simulink model "satellite3"  (R2025b)
settings: Solver=FixedStepAuto  StartTime=0.0  StopTime=100  FixedStep=dt  MinStep=0.0001  RelTol=1e-3
values from neighbouring files (symbols this model uses):
  A_mw = [ ... (first row only)    [init_params.m]
  A_w = [ ... (first row only)    [init_params.m]
  alpha1 = 0.1    [init_params.m]
  alpha2 = 0.1    [init_params.m]
  angle0 = eAR'    [init_params.m]
  area_d = 4    [init_params.m]
  area_m2 = 0.0127    [init_params.m]
  area_s = 2    [init_params.m]
  ARW_deg_per_sqrt_h = 0.01    [init_params.m]
  B_mw = [ ... (first row only)    [init_params.m]
  bat_bias_on = 0    [init_params.m]
  bat_bias_time = 0    [init_params.m]
  bat_bias_value = 0    [init_params.m]
  bat_cap_on = 0    [init_params.m]
  bat_cap_time = 0    [init_params.m]
  bat_cap_value = 1    [init_params.m]
  beta = 0.3    [init_params.m]
  beta1 = 0.01    [init_params.m]
  beta2 = 0.01    [init_params.m]
  bias0_deg_h = 0.01    [init_params.m]
  C_mw = [ ... (first row only)    [init_params.m]
  Cd = 2.2    [init_params.m]
  Cm = 0.01    [init_params.m]
  cmd_comm = 1    [init_params.m]
  comm_allow = 1    [init_params.m]
  cos_g_max = cos(gamma_max)    [init_params.m]
  Cr = 1.2    [init_params.m]
  cT_deg_on = 0    [init_params.m]
  cT_deg_time = 0    [init_params.m]
  cT_deg_value = 1    [init_params.m]
  cT_delay_on = 0    [init_params.m]
  cT_delay_time = 0    [init_params.m]
  cT_delay_value = 0    [init_params.m]
  cT_drop_on = 0    [init_params.m]
  cT_drop_time = 0    [init_params.m]
  cT_drop_value = 0    [init_params.m]
  cT_lock_on = 0    [init_params.m]
  cT_lock_time = 0    [init_params.m]
  d_c = 2e-5    (= 2e-05)    [init_params.m]
  d_f = 2e-5    (= 2e-05)    [init_params.m]
  D_max = 1    [init_params.m]
  D_thr = 0.4    [init_params.m]
  Delta_D = 0.001    [init_params.m]
  dP_th = 0.05    [init_params.m]
  dss_bias_on = 0    [init_params.m]
  dss_bias_time = 0    [init_params.m]
  dss_bias_value = [0;0;0]    [init_params.m]
  dss_delay_on = 0    [init_params.m]
  dss_delay_time = 0    [init_params.m]
  dss_delay_value = 0    [init_params.m]
  dss_drift_max = 0.1    [init_params.m]
  dss_drift_value = [0;0;0]    [init_params.m]
  dss_drop_on = 0    [init_params.m]
  dss_drop_time = 0    [init_params.m]
  dss_drop_value = [1;0;0]    [init_params.m]
  dss_lock_on = 0    [init_params.m]
  dss_lock_time = 0    [init_params.m]
  dt = 0.1    [init_params.m]
  earth_theta0 = 0    [init_params.m]
  epsilon = 0.01    [init_params.m]
  eT_deg_on = 0    [init_params.m]
  eT_deg_time = 0    [init_params.m]
  eT_deg_value = 1    [init_params.m]
  eT_delay_on = 0    [init_params.m]
  eT_delay_time = 0    [init_params.m]
  eT_delay_value = 0    [init_params.m]
  eT_drop_on = 0    [init_params.m]
  eT_drop_time = 0    [init_params.m]
  eT_drop_value = [0;0;0]    [init_params.m]
  eT_lock_on = 0    [init_params.m]
  eT_lock_time = 0    [init_params.m]
  eta = 0.7    [init_params.m]
  eta_buck = 0.9    [init_params.m]
  eta_et = 0.9    [init_params.m]
  eta_sspa = 0.35    [init_params.m]
  eta_twta = 0.35    [init_params.m]
  f = 2.2e9    (= 2200000000)    [init_params.m]
  f_n_hz = 400    [init_params.m]
  fov = 60*pi/180    (= 1.0471975512)    [init_params.m]
  g0 = 9.80665    [init_params.m]
  G0 = 1366.1    [init_params.m]
  G_sspa_dB = 20    [init_params.m]
  G_twta_dB = 20    [init_params.m]
  Gr_dB = 20    [init_params.m]
  Gt_dB = 3    [init_params.m]
  gyro_bias_on = 0    [init_params.m]
  gyro_bias_time = 0    [init_params.m]
  gyro_bias_value = [0;0;0]    [init_params.m]
  gyro_delay_on = 0    [init_params.m]
  gyro_delay_time = 0    [init_params.m]
  gyro_delay_value = 0    [init_params.m]
  gyro_drift_max = 0.1    [init_params.m]
  gyro_drift_value = [0;0;0]    [init_params.m]
  gyro_drop_on = 0    [init_params.m]
  gyro_drop_time = 0    [init_params.m]
  gyro_drop_value = [0;0;0]    [init_params.m]
  gyro_lock_on = 0    [init_params.m]
  gyro_lock_time = 0    [init_params.m]
  H = 50e3    (= 50000)    [init_params.m]
  h_max = Iw * rpm_max * sqrt(6)    [init_params.m]
  h_ref = 400e3    (= 400000)    [init_params.m]
  I_e = 11    [init_params.m]
  I_gate = 0.5    [init_params.m]
  I_triggle = 8    [init_params.m]
  i_w_max = 2    [init_params.m]
  i_w_min = -2    [init_params.m]
  initial_phase = 0    [init_params.m]
  Isp = 220    [init_params.m]
  Isp_et = 1500    [init_params.m]
  Iw = 0.02    [init_params.m]
  J2 = 1.08262668e-3    (= 0.00108262668)    [init_params.m]
  Jx = 10    [init_params.m]
  Jy = 12    [init_params.m]
  Jz = 8    [init_params.m]
  k_a = 4e-4    (= 0.0004)    [init_params.m]
  k_bias1_deg_h_per_C = 1    [init_params.m]
  k_bias2_deg_h_per_C = 0.0    (= 0)    [init_params.m]
  k_h = -0.05    [init_params.m]
  k_sf1_ppm = 1.0    (= 1)    [init_params.m]
  k_sf2_ppm = 0.0    (= 0)    [init_params.m]
  ... (+207 more)
libraries: matrix_library x25, simulink x14, nesl_utility x4, simulink_extras x3, fl_lib x3, ee_lib x1
(part 4 of 5)

== system satellite3/姿态确定与控制系统/三轴姿态动力学子系统/姿态解算/简化互补滤波器/四元数乘法 ==
  Q1 : Inport
  Q2 : Inport  Port=2
  Add : Sum  Inputs=3
  Cross Product : matrix_library/Cross Product
  Demux : Demux
  Demux1 : Demux
  Dot Product : DotProduct  OutDataTypeStr=Inherit: Inherit via internal rule
  Mux : Mux  Inputs=2
  Mux1 : Mux  Inputs=3
  Mux2 : Mux  Inputs=3
  Product : Product
  Product1 : Product
  Product2 : Product
  Sum : Sum  Inputs=|+-
  Q : Outport
  wires:
  Q1/1 -> Demux/1
  Q2/1 -> Demux1/1
  Mux/1 -> Q/1
  Product/1 -> Sum/1
  Demux/1 -> Product1/1, Product/1
  Mux1/1 -> Dot Product/1, Cross Product/1, Product2/2
  Demux1/1 -> Product2/1, Product/2
  Mux2/1 -> Cross Product/2, Dot Product/2, Product1/2
  Sum/1 -> Mux/1
  Dot Product/1 -> Sum/2
  Product2/1 -> Add/2
  Product1/1 -> Add/1
  Cross Product/1 -> Add/3
  Add/1 -> Mux/2
  Demux/2 -> Mux1/1
  Demux/3 -> Mux1/2
  Demux/4 -> Mux1/3
  Demux1/2 -> Mux2/1
  Demux1/3 -> Mux2/2
  Demux1/4 -> Mux2/3

== system satellite3/姿态确定与控制系统/三轴姿态动力学子系统/姿态解算/简化互补滤波器/四元数传播-欧拉法 ==
  note: $\dot{q}=\frac{1}{2} \left[\begin{array}{ccc} -q_1&-q_2&-q_3 \\ q_0&-q_3&q_2\\ q_3&q_0&-q_1\\ -q_2&q_1&q_0 \end{array}\right]\omega$
  机体系角速度分量 : Inport
  Demux : Demux
  Int_q0 : Integrator  InitialCondition=Q0(1)
  Int_q1 : Integrator  InitialCondition=Q0(2)
  Int_q2 : Integrator  InitialCondition=Q0(3)
  Int_q3 : Integrator  InitialCondition=Q0(4)
  Mux : Mux
  Product : Product  Multiplication=Matrix(*)
  Product{1..4} (4 alike) : Product  Inputs=*/
  Transpose : Math  Operator=transpose
  Vector Concatenate : Concatenate  NumInputs=4  Mode=Multidimensional array  ConcatenateDimension=2
  neg1 : Gain  Gain=-1
  neg2 : Gain  Gain=-1
  neg3 : Gain  Gain=-1
  q0_dot : Mux  Inputs=3
  q1_dot : Mux  Inputs=3
  q1_dot1 : Mux  Inputs=3
  q1_dot2 : Mux  Inputs=3
  向量模长-q : Subsystem
  四元数 : Outport
  wires:
  Product/1 -> Demux/1
  neg1/1 -> q0_dot/1, q1_dot1/3
  q1_dot/1 -> Vector Concatenate/2
  neg3/1 -> q1_dot/2, q0_dot/3
  Product4/1 -> neg3/1, Mux/4, q1_dot1/1  "q3"
  Product1/1 -> q1_dot/1, q1_dot1/2, Mux/1, q1_dot2/3  "q0"
  q1_dot1/1 -> Vector Concatenate/3
  Demux/2 -> Int_q1/1
  Product2/1 -> neg1/1, Mux/2, q1_dot2/2  "q1"
  Demux/3 -> Int_q2/1
  neg2/1 -> q1_dot2/1, q0_dot/2
  q1_dot2/1 -> Vector Concatenate/4
  Product3/1 -> neg2/1, Mux/3, q1_dot/3  "q2"
  q0_dot/1 -> Vector Concatenate/1
  Vector Concatenate/1 -> Transpose/1
  Demux/1 -> Int_q0/1
  Demux/4 -> Int_q3/1
  机体系角速度分量/1 -> Product/2
  Transpose/1 -> Product/1
  Int_q0/1 -> Product1/1, 向量模长-q/1(u0)
  Int_q1/1 -> Product2/1, 向量模长-q/2(u1)
  Int_q2/1 -> Product3/1, 向量模长-q/3(u2)
  Int_q3/1 -> Product4/1, 向量模长-q/4(u3)
  向量模长-q/1(|u|) -> Product2/2, Product3/2, Product4/2, Product1/2
  Mux/1 -> 四元数/1

== system satellite3/姿态确定与控制系统/三轴姿态动力学子系统/姿态解算/简化互补滤波器/太敏&地敏 ==
  note: 可见性：一般只要不被遮挡都能工作；
      | 当高度太高（或地球在传感器背面）判 invalid
  太阳矢量 : Inport
  hat_r_o : Inport  Port=2
  q_hat : Inport  Port=3
  q_true : Inport  Port=4
  Add : Sum
  Cross Product : matrix_library/Cross Product
  Cross Product1 : matrix_library/Cross Product
  Gain : Gain  Gain=0.6
  Gain1 : Gain  Gain=0.4
  地敏测量 : Subsystem
  地敏预测 : Subsystem
  太敏测量 : Subsystem
  太敏预测 : Subsystem
  e_c : Outport
  wires:
  太阳矢量/1 -> 太敏测量/2(太阳矢量), 太敏预测/2(太阳矢量)
  hat_r_o/1 -> 地敏预测/1(hat_r_o), 地敏测量/1(hat_r_o)
  太敏预测/1(s_b_meas) -> Cross Product/1
  太敏测量/1(s_b_meas) -> Cross Product/2
  q_true/1 -> 地敏测量/2(q_true), 太敏测量/1(q_true)
  q_hat/1 -> 太敏预测/1(q_hat), 地敏预测/3(q_hat)
  地敏预测/1(nadir_b_meas) -> Cross Product1/1
  地敏测量/1(nadir_b_meas) -> Cross Product1/2
  Cross Product/1 -> Gain/1
  Cross Product1/1 -> Gain1/1
  Gain/1 -> Add/1
  Gain1/1 -> Add/2
  Add/1 -> e_c/1

== system satellite3/姿态确定与控制系统/三轴姿态动力学子系统/姿态解算/简化互补滤波器/星敏故障 ==
  原值 : Inport
  Add : Sum  Inputs=+++++
  Sum : Sum  Inputs=|++
  偏差故障 : Subsystem
  延迟故障 : Subsystem
  掉线故障 : Subsystem
  漂移故障 : Subsystem
  锁死故障 : Subsystem
  故障值 : Outport
  wires:
  延迟故障/1(故障值注入) -> Add/5
  掉线故障/1(故障值注入) -> Add/4
  锁死故障/1(故障值注入) -> Add/3
  漂移故障/1(故障值注入) -> Add/2
  偏差故障/1(故障值注入) -> Add/1
  Add/1 -> Sum/2
  Sum/1 -> 故障值/1
  原值/1 -> Sum/1, 锁死故障/1(原值), 掉线故障/1(原值), 延迟故障/1(原值)

== system satellite3/姿态确定与控制系统/金字塔反作用轮组件/反作用轮组件/反作用轮1/摩擦模型 ==
  note: Stribeck/死区/轴承复杂摩擦:是真实工程里会做的，但不建议上。因为：
      | 参数难找
      | 容易导致数值振荡
      | 对系统级闭环验证意义不如前两层大
  转速 : Inport
  Add : Sum
  Sign : Signum
  库仑摩擦系数 : Gain  Gain=d_c
  粘性摩擦系数 : Gain  Gain=d_f
  摩擦力矩 : Outport
  wires:
  转速/1 -> 粘性摩擦系数/1, Sign/1
  Sign/1 -> 库仑摩擦系数/1
  库仑摩擦系数/1 -> Add/2
  粘性摩擦系数/1 -> Add/1
  Add/1 -> 摩擦力矩/1

== system satellite3/姿态确定与控制系统/金字塔反作用轮组件/反作用轮组件/反作用轮1/轮力矩故障 ==
  原值 : Inport
  Add : Sum  Inputs=++++++
  Sum : Sum  Inputs=|++
  延迟故障 : Subsystem
  掉线故障 : Subsystem
  迟缓故障 : Subsystem
  退化故障 : Subsystem
  锁死故障 : Subsystem
  饱和故障 : Subsystem
  故障值 : Outport
  wires:
  延迟故障/1(故障值注入) -> Add/3
  饱和故障/1(故障值注入) -> Add/2
  退化故障/1(故障值注入) -> Add/1
  Add/1 -> Sum/2
  Sum/1 -> 故障值/1
  原值/1 -> Sum/1, 锁死故障/1(原值), 迟缓故障/1(原值), 掉线故障/1(原值), 延迟故障/1(原值), 饱和故障/1(原值), 退化故障/1(原值)
  掉线故障/1(故障值注入) -> Add/4
  迟缓故障/1(故障值注入) -> Add/5
  锁死故障/1(故障值注入) -> Add/6

== system satellite3/姿态确定与控制系统/金字塔反作用轮组件/反作用轮组件/反作用轮1/轮摩擦故障 ==
  原值 : Inport
  Add : Sum
  Sum : Sum  Inputs=|++
  乘性故障 : Subsystem
  偏差故障 : Subsystem
  故障值 : Outport
  wires:
  乘性故障/1(故障值注入) -> Add/2
  Sum/1 -> 故障值/1
  原值/1 -> Sum/1, 乘性故障/1(原值)
  偏差故障/1(故障值注入) -> Add/1
  Add/1 -> Sum/2

== system satellite3/姿态确定与控制系统/金字塔反作用轮组件/反作用轮组件/反作用轮1/轮状态解算 ==
  作用力矩 : Inport
  积分得到转速 : Integrator
  转动惯量 : Gain  Gain=Iw
  除以转动惯量 : Gain  Gain=1/Iw
  转速 : Outport
  角动量 : Outport  Port=2
  wires:
  积分得到转速/1 -> 转动惯量/1, 转速/1
  除以转动惯量/1 -> 积分得到转速/1
  作用力矩/1 -> 除以转动惯量/1
  转动惯量/1 -> 角动量/1

== system satellite3/姿态确定与控制系统/金字塔反作用轮组件/反作用轮组件/反作用轮2/摩擦模型 ==
  note: Stribeck/死区/轴承复杂摩擦:是真实工程里会做的，但不建议上。因为：
      | 参数难找
      | 容易导致数值振荡
      | 对系统级闭环验证意义不如前两层大
  转速 : Inport
  Add : Sum
  Sign : Signum
  库仑摩擦系数 : Gain  Gain=d_c
  粘性摩擦系数 : Gain  Gain=d_f
  摩擦力矩 : Outport
  wires:
  Add/1 -> 摩擦力矩/1
  粘性摩擦系数/1 -> Add/1
  库仑摩擦系数/1 -> Add/2
  Sign/1 -> 库仑摩擦系数/1
  转速/1 -> Sign/1, 粘性摩擦系数/1

== system satellite3/姿态确定与控制系统/金字塔反作用轮组件/反作用轮组件/反作用轮2/轮力矩故障 ==
  原值 : Inport
  Add : Sum  Inputs=++++++
  Sum : Sum  Inputs=|++
  延迟故障 : Subsystem
  掉线故障 : Subsystem
  迟缓故障 : Subsystem
  退化故障 : Subsystem
  锁死故障 : Subsystem
  饱和故障 : Subsystem
  故障值 : Outport
  wires:
  锁死故障/1(故障值注入) -> Add/6
  迟缓故障/1(故障值注入) -> Add/5
  掉线故障/1(故障值注入) -> Add/4
  原值/1 -> 退化故障/1(原值), 饱和故障/1(原值), 延迟故障/1(原值), 掉线故障/1(原值), 迟缓故障/1(原值), 锁死故障/1(原值), Sum/1
  Sum/1 -> 故障值/1
  Add/1 -> Sum/2
  退化故障/1(故障值注入) -> Add/1
  饱和故障/1(故障值注入) -> Add/2
  延迟故障/1(故障值注入) -> Add/3

== system satellite3/姿态确定与控制系统/金字塔反作用轮组件/反作用轮组件/反作用轮2/轮摩擦故障 ==
  原值 : Inport
  Add : Sum
  Sum : Sum  Inputs=|++
  乘性故障 : Subsystem
  偏差故障 : Subsystem
  故障值 : Outport
  wires:
  乘性故障/1(故障值注入) -> Add/2
  Sum/1 -> 故障值/1
  原值/1 -> Sum/1, 乘性故障/1(原值)
  偏差故障/1(故障值注入) -> Add/1
  Add/1 -> Sum/2

== system satellite3/姿态确定与控制系统/金字塔反作用轮组件/反作用轮组件/反作用轮2/轮状态解算 ==
  作用力矩 : Inport
  积分得到转速 : Integrator
  转动惯量 : Gain  Gain=Iw
  除以转动惯量 : Gain  Gain=1/Iw
  转速 : Outport
  角动量 : Outport  Port=2
  wires:
  转动惯量/1 -> 角动量/1
  作用力矩/1 -> 除以转动惯量/1
  除以转动惯量/1 -> 积分得到转速/1
  积分得到转速/1 -> 转速/1, 转动惯量/1

== system satellite3/姿态确定与控制系统/金字塔反作用轮组件/反作用轮组件/反作用轮3/摩擦模型 ==
  note: Stribeck/死区/轴承复杂摩擦:是真实工程里会做的，但不建议上。因为：
      | 参数难找
      | 容易导致数值振荡
      | 对系统级闭环验证意义不如前两层大
  转速 : Inport
  Add : Sum
  Sign : Signum
  库仑摩擦系数 : Gain  Gain=d_c
  粘性摩擦系数 : Gain  Gain=d_f
  摩擦力矩 : Outport
  wires:
  转速/1 -> 粘性摩擦系数/1, Sign/1
  Sign/1 -> 库仑摩擦系数/1
  库仑摩擦系数/1 -> Add/2
  粘性摩擦系数/1 -> Add/1
  Add/1 -> 摩擦力矩/1

== system satellite3/姿态确定与控制系统/金字塔反作用轮组件/反作用轮组件/反作用轮3/轮力矩故障 ==
  原值 : Inport
  Add : Sum  Inputs=++++++
  Sum : Sum  Inputs=|++
  延迟故障 : Subsystem
  掉线故障 : Subsystem
  迟缓故障 : Subsystem
  退化故障 : Subsystem
  锁死故障 : Subsystem
  饱和故障 : Subsystem
  故障值 : Outport
  wires:
  延迟故障/1(故障值注入) -> Add/3
  饱和故障/1(故障值注入) -> Add/2
  退化故障/1(故障值注入) -> Add/1
  Add/1 -> Sum/2
  Sum/1 -> 故障值/1
  原值/1 -> Sum/1, 锁死故障/1(原值), 迟缓故障/1(原值), 掉线故障/1(原值), 延迟故障/1(原值), 饱和故障/1(原值), 退化故障/1(原值)
  掉线故障/1(故障值注入) -> Add/4
  迟缓故障/1(故障值注入) -> Add/5
  锁死故障/1(故障值注入) -> Add/6

== system satellite3/姿态确定与控制系统/金字塔反作用轮组件/反作用轮组件/反作用轮3/轮摩擦故障 ==
  原值 : Inport
  Add : Sum
  Sum : Sum  Inputs=|++
  乘性故障 : Subsystem
  偏差故障 : Subsystem
  故障值 : Outport
  wires:
  乘性故障/1(故障值注入) -> Add/2
  Sum/1 -> 故障值/1
  原值/1 -> Sum/1, 乘性故障/1(原值)
  偏差故障/1(故障值注入) -> Add/1
  Add/1 -> Sum/2

== system satellite3/姿态确定与控制系统/金字塔反作用轮组件/反作用轮组件/反作用轮3/轮状态解算 ==
  作用力矩 : Inport
  积分得到转速 : Integrator
  转动惯量 : Gain  Gain=Iw
  除以转动惯量 : Gain  Gain=1/Iw
  转速 : Outport
  角动量 : Outport  Port=2
  wires:
  积分得到转速/1 -> 转动惯量/1, 转速/1
  除以转动惯量/1 -> 积分得到转速/1
  作用力矩/1 -> 除以转动惯量/1
  转动惯量/1 -> 角动量/1

== system satellite3/姿态确定与控制系统/金字塔反作用轮组件/反作用轮组件/反作用轮4/摩擦模型 ==
  note: Stribeck/死区/轴承复杂摩擦:是真实工程里会做的，但不建议上。因为：
      | 参数难找
      | 容易导致数值振荡
      | 对系统级闭环验证意义不如前两层大
  转速 : Inport
  Add : Sum
  Sign : Signum
  库仑摩擦系数 : Gain  Gain=d_c
  粘性摩擦系数 : Gain  Gain=d_f
  摩擦力矩 : Outport
  wires:
  Add/1 -> 摩擦力矩/1
  粘性摩擦系数/1 -> Add/1
  库仑摩擦系数/1 -> Add/2
  Sign/1 -> 库仑摩擦系数/1
  转速/1 -> Sign/1, 粘性摩擦系数/1

== system satellite3/姿态确定与控制系统/金字塔反作用轮组件/反作用轮组件/反作用轮4/轮力矩故障 ==
  原值 : Inport
  Add : Sum  Inputs=++++++
  Sum : Sum  Inputs=|++
  延迟故障 : Subsystem
  掉线故障 : Subsystem
  迟缓故障 : Subsystem
  退化故障 : Subsystem
  锁死故障 : Subsystem
  饱和故障 : Subsystem
  故障值 : Outport
  wires:
  锁死故障/1(故障值注入) -> Add/6
  迟缓故障/1(故障值注入) -> Add/5
  掉线故障/1(故障值注入) -> Add/4
  原值/1 -> 退化故障/1(原值), 饱和故障/1(原值), 延迟故障/1(原值), 掉线故障/1(原值), 迟缓故障/1(原值), 锁死故障/1(原值), Sum/1
  Sum/1 -> 故障值/1
  Add/1 -> Sum/2
  退化故障/1(故障值注入) -> Add/1
  饱和故障/1(故障值注入) -> Add/2
  延迟故障/1(故障值注入) -> Add/3

== system satellite3/姿态确定与控制系统/金字塔反作用轮组件/反作用轮组件/反作用轮4/轮摩擦故障 ==
  原值 : Inport
  Add : Sum
  Sum : Sum  Inputs=|++
  乘性故障 : Subsystem
  偏差故障 : Subsystem
  故障值 : Outport
  wires:
  乘性故障/1(故障值注入) -> Add/2
  Sum/1 -> 故障值/1
  原值/1 -> Sum/1, 乘性故障/1(原值)
  偏差故障/1(故障值注入) -> Add/1
  Add/1 -> Sum/2

== system satellite3/姿态确定与控制系统/金字塔反作用轮组件/反作用轮组件/反作用轮4/轮状态解算 ==
  作用力矩 : Inport
  积分得到转速 : Integrator
  转动惯量 : Gain  Gain=Iw
  除以转动惯量 : Gain  Gain=1/Iw
  转速 : Outport
  角动量 : Outport  Port=2
  wires:
  转动惯量/1 -> 角动量/1
  作用力矩/1 -> 除以转动惯量/1
  除以转动惯量/1 -> 积分得到转速/1
  积分得到转速/1 -> 转速/1, 转动惯量/1

== system satellite3/电源子系统/太阳能板/太阳板/伏电特性/Sensing Current ==
  Current Sensor : fl_lib/Electrical/Electrical Sensors/Current Sensor
  PS-Simulink/I : nesl_utility/PS-Simulink Converter  PhysicalDomain=network_engine_domain  SubClassName=ps_output  LeftPortType=input  RightPortType=output  PseudoPeriodic=off  Frequencies=[]  VectorFormat=1-D array  Unit=1  AffineConversion=off
  Conn1 : PMIOPort  Side=Left
  Conn2 : PMIOPort  Port=2  Side=Right
  Out1 : Outport  VectorParamsAs1DForOutWhenUnconnected=off
  wires:
  PS-Simulink/I/1 -> Out1/1
  connections:
  Current Sensor/RConn1 -- PS-Simulink/I/LConn1
  Current Sensor/LConn1 -- Conn1/RConn1
  Conn2/RConn1 -- Current Sensor/RConn2

== system satellite3/电源子系统/太阳能板/太阳板/入射角余弦/余弦夹角 ==
  u1 : Inport
  u2 : Inport  Port=2
  Demux : Demux  Outputs=3
  Demux1 : Demux  Outputs=3
  Dot Product : DotProduct  OutDataTypeStr=Inherit: Inherit via internal rule
  余弦夹角 : Product  Inputs=/*/
  向量模长-r1 : Subsystem
  向量模长-r2 : Subsystem
  cos(γ) : Outport
  wires:
  向量模长-r2/1(|u|) -> 余弦夹角/3
  Demux/3 -> 向量模长-r1/3(u3)
  Demux/2 -> 向量模长-r1/2(u2)
  Dot Product/1 -> 余弦夹角/2
  Demux/1 -> 向量模长-r1/1(u1)
  向量模长-r1/1(|u|) -> 余弦夹角/1
  u2/1 -> Dot Product/2, Demux1/1
  Demux1/1 -> 向量模长-r2/1(u1)
  Demux1/2 -> 向量模长-r2/2(u2)
  Demux1/3 -> 向量模长-r2/3(u3)
  u1/1 -> Dot Product/1, Demux/1
  余弦夹角/1 -> cos(γ)/1

== system satellite3/电源子系统/太阳能板/太阳板/入射角余弦/共轭 ==
  q : Inport
  -qd1 : Gain  Gain=-1
  -qd2 : Gain  Gain=-1
  -qd3 : Gain  Gain=-1
  Demux : Demux
  Mux : Mux
  q* : Outport
  wires:
  q/1 -> Demux/1
  Mux/1 -> q*/1
  Demux/1 -> Mux/1
  Demux/2 -> -qd1/1
  -qd1/1 -> Mux/2
  Demux/3 -> -qd2/1
  -qd2/1 -> Mux/3
  Demux/4 -> -qd3/1
  -qd3/1 -> Mux/4

== system satellite3/电源子系统/太阳能板/太阳板/入射角余弦/四元数乘法 ==
  Q1 : Inport
  Q2 : Inport  Port=2
  Add : Sum  Inputs=3
  Cross Product : matrix_library/Cross Product
  Demux : Demux
  Demux1 : Demux
  Dot Product : DotProduct  OutDataTypeStr=Inherit: Inherit via internal rule
  Mux : Mux  Inputs=2
  Mux1 : Mux  Inputs=3
  Mux2 : Mux  Inputs=3
  Product : Product
  Product1 : Product
  Product2 : Product
  Sum : Sum  Inputs=|+-
  Q* : Outport
  wires:
  Q1/1 -> Demux/1
  Q2/1 -> Demux1/1
  Mux/1 -> Q*/1
  Product/1 -> Sum/1
  Demux/1 -> Product1/1, Product/1
  Mux1/1 -> Dot Product/1, Cross Product/1, Product2/2
  Demux1/1 -> Product2/1, Product/2
  Mux2/1 -> Cross Product/2, Dot Product/2, Product1/2
  Sum/1 -> Mux/1
  Dot Product/1 -> Sum/2
  Product2/1 -> Add/2
  Product1/1 -> Add/1
  Cross Product/1 -> Add/3
  Add/1 -> Mux/2
  Demux/2 -> Mux1/1
  Demux/3 -> Mux1/2
  Demux/4 -> Mux1/3
  Demux1/2 -> Mux2/1
  Demux1/3 -> Mux2/2
  Demux1/4 -> Mux2/3

== system satellite3/电源子系统/太阳能板/太阳板/入射角余弦/四元数旋转 ==
  Q1 : Inport
  Q2 : Inport  Port=2
  Add : Sum  Inputs=3
  Cross Product : matrix_library/Cross Product
  Demux : Demux
  Demux1 : Demux
  Mux1 : Mux  Inputs=3
  Mux2 : Mux  Inputs=3
  Product1 : Product
  Product2 : Product
  Q* : Outport
  wires:
  Demux1/4 -> Mux2/3
  Demux1/3 -> Mux2/2
  Demux1/2 -> Mux2/1
  Demux/4 -> Mux1/3
  Demux/3 -> Mux1/2
  Demux/2 -> Mux1/1
  Add/1 -> Q*/1
  Cross Product/1 -> Add/3
  Product1/1 -> Add/1
  Product2/1 -> Add/2
  Mux2/1 -> Product1/2, Cross Product/2
  Demux1/1 -> Product2/1
  Mux1/1 -> Product2/2, Cross Product/1
  Demux/1 -> Product1/1
  Q2/1 -> Demux1/1
  Q1/1 -> Demux/1

== system satellite3/电源子系统/太阳能板/太阳板/太阳翼故障/掉线故障 ==
  原值 : Inport
  Switch : Switch  Criteria=u2 > Threshold  Threshold=0.5  SaturateOnIntegerOverflow=off  InputSameDT=off
  Zero : Constant  Value=wing_drop_value  OutDataTypeStr=Inherit: Inherit via back propagation
  使能 : Gain  Gain=wing_drop_on
  抵消 : Sum  Inputs=|+-
  注入时间 : Step  Time=wing_drop_time  SampleTime=0
  故障值注入 : Outport
  wires:
  使能/1 -> Switch/2
  注入时间/1 -> 使能/1
  原值/1 -> Switch/3, 抵消/2
  抵消/1 -> 故障值注入/1
  Switch/1 -> 抵消/1
  Zero/1 -> Switch/1

== system satellite3/电源子系统/太阳能板/太阳板/太阳翼故障/退化故障 ==
  原值 : Inport
  Switch : Switch  Criteria=u2 > Threshold  Threshold=0.5  SaturateOnIntegerOverflow=off  InputSameDT=off
  使能 : Gain  Gain=wing_deg_on
  幅度 : Gain  Gain=wing_deg_value
  抵消 : Sum  Inputs=|+-
  注入时间 : Step  Time=wing_deg_time  SampleTime=0
  故障值注入 : Outport
  wires:
  Switch/1 -> 抵消/1
  原值/1 -> 抵消/2, 幅度/1, Switch/3
  使能/1 -> Switch/2
  抵消/1 -> 故障值注入/1
  注入时间/1 -> 使能/1
  幅度/1 -> Switch/1

== system satellite3/姿态确定与控制系统/三轴姿态动力学子系统/姿态解算/星敏/四元数归一化/向量模长-q ==
  u0 : Inport
  u1 : Inport  Port=2
  u2 : Inport  Port=3
  u3 : Inport  Port=4
  Add : Sum  Inputs=4
  Sqrt : Sqrt
  Square{,1..3} (4 alike) : Math  Operator=square
  |u| : Outport
  wires:
  u0/1 -> Square/1
  u1/1 -> Square1/1
  u2/1 -> Square2/1
  Square/1 -> Add/1
  Square1/1 -> Add/2
  Square2/1 -> Add/3
  Add/1 -> Sqrt/1
  Sqrt/1 -> |u|/1
  u3/1 -> Square3/1
  Square3/1 -> Add/4

== system satellite3/姿态确定与控制系统/三轴姿态动力学子系统/姿态解算/简化互补滤波器/四元数传播-欧拉法/向量模长-q ==
  u0 : Inport
  u1 : Inport  Port=2
  u2 : Inport  Port=3
  u3 : Inport  Port=4
  Add : Sum  Inputs=4
  Sqrt : Sqrt
  Square{,1..3} (4 alike) : Math  Operator=square
  |u| : Outport
  wires:
  u0/1 -> Square/1
  u1/1 -> Square1/1
  u2/1 -> Square2/1
  Square/1 -> Add/1
  Square1/1 -> Add/2
  Square2/1 -> Add/3
  Add/1 -> Sqrt/1
  Sqrt/1 -> |u|/1
  u3/1 -> Square3/1
  Square3/1 -> Add/4

== system satellite3/姿态确定与控制系统/三轴姿态动力学子系统/姿态解算/简化互补滤波器/太敏&地敏/地敏测量 ==
  note: 地敏通常测地球地平线，用于粗地心指向。工程等效可以用“地心方向”来代表它输出的姿态信息
  hat_r_o : Inport
  q_true : Inport  Port=2
  Demux2 : Demux  Outputs=3
  Divide : Product  Inputs=*/
  Mux : Mux  Inputs=2
  hat-s_b : Subsystem
  共轭 : Subsystem
  向量模长-s_b : Subsystem
  四元数乘法 : Subsystem
  nadir_b_meas : Outport
  wires:
  Demux2/1 -> 向量模长-s_b/1(u0)
  hat-s_b/1(hat_r_b) -> Divide/1, Demux2/1
  [zero] -> Mux/1
  q_true/1 -> hat-s_b/2(Q2), 共轭/1(q)
  共轭/1(q*) -> 四元数乘法/1(Q1)
  hat_r_o/1 -> Mux/2
  Mux/1 -> 四元数乘法/2(Q2)
  四元数乘法/1(Q*) -> hat-s_b/1(Q1)
  Demux2/2 -> 向量模长-s_b/2(u1)
  Demux2/3 -> 向量模长-s_b/3(u2)
  向量模长-s_b/1(|u|) -> Divide/2
  Divide/1 -> nadir_b_meas/1

== system satellite3/姿态确定与控制系统/三轴姿态动力学子系统/姿态解算/简化互补滤波器/太敏&地敏/地敏预测 ==
  note: 地敏通常测地球地平线，用于粗地心指向。工程等效可以用“地心方向”来代表它输出的姿态信息
  hat_r_o : Inport
  valid : Inport  Port=2
  q_hat : Inport  Port=3
  Add : Sum
  Demux2 : Demux  Outputs=3
  Divide : Product  Inputs=*/
  Mux : Mux  Inputs=2
  hat-s_b : Subsystem
  hat_b_r : Gain  Gain=-1
  共轭 : Subsystem
  向量模长-s_b : Subsystem
  四元数乘法 : Subsystem
  地敏噪声 : Subsystem
  nadir_b_meas : Outport
  wires:
  hat_b_r/1 -> Add/1
  地敏噪声/1(noise) -> Add/2
  Demux2/2 -> 向量模长-s_b/2(u1)
  向量模长-s_b/1(|u|) -> Divide/2
  Demux2/1 -> 向量模长-s_b/1(u0)
  Add/1 -> Divide/1, Demux2/1
  Demux2/3 -> 向量模长-s_b/3(u2)
  Divide/1 -> nadir_b_meas/1
  共轭/1(q*) -> 四元数乘法/1(Q1)
  Mux/1 -> 四元数乘法/2(Q2)
  [zero] -> Mux/1
  q_hat/1 -> hat-s_b/2(Q2), 共轭/1(q)
  四元数乘法/1(Q*) -> hat-s_b/1(Q1)
  hat_r_o/1 -> Mux/2
  hat-s_b/1(hat_r_b) -> hat_b_r/1

== system satellite3/姿态确定与控制系统/三轴姿态动力学子系统/姿态解算/简化互补滤波器/太敏&地敏/太敏测量 ==
  q_true : Inport
  太阳矢量 : Inport  Port=2
  Demux2 : Demux  Outputs=3
  Divide : Product  Inputs=*/
  Mux : Mux  Inputs=2
  hat-s_b : Subsystem
  共轭 : Subsystem
  向量模长-s_b : Subsystem
  四元数乘法 : Subsystem
  s_b_meas : Outport
  wires:
  共轭/1(q*) -> 四元数乘法/1(Q1)
  [zero] -> Mux/1
  Demux2/1 -> 向量模长-s_b/1(u0)
  hat-s_b/1(Q*) -> Divide/1, Demux2/1
  q_true/1 -> hat-s_b/2(Q2), 共轭/1(q)
  四元数乘法/1(Q*) -> hat-s_b/1(Q1)
  Mux/1 -> 四元数乘法/2(Q2)
  太阳矢量/1 -> Mux/2
  Demux2/2 -> 向量模长-s_b/2(u1)
  Demux2/3 -> 向量模长-s_b/3(u2)
  向量模长-s_b/1(|u|) -> Divide/2
  Divide/1 -> s_b_meas/1

== system satellite3/姿态确定与控制系统/三轴姿态动力学子系统/姿态解算/简化互补滤波器/太敏&地敏/太敏预测 ==
  q_hat : Inport
  太阳矢量 : Inport  Port=2
  Add : Sum
  Constant : Constant  Value=n_sun
  Constant1 : Constant  Value=cos(fov)
  Demux2 : Demux  Outputs=3
  Divide : Product  Inputs=*/
  Dot Product : DotProduct  OutDataTypeStr=Inherit: Inherit via internal rule
  Mux : Mux  Inputs=2
  Relational Operator : RelationalOperator  Operator=>  OutDataTypeStr=boolean  RndMeth=Simplest  InputSameDT=off
  hat-s_b : Subsystem
  共轭 : Subsystem
  向量模长-s_b : Subsystem
  四元数乘法 : Subsystem
  太敏噪声 : Subsystem
  太敏故障 : Subsystem
  s_b_meas : Outport
  valid : Outport  Port=2
  wires:
  太阳矢量/1 -> Mux/2
  [zero] -> Mux/1
  q_hat/1 -> hat-s_b/2(Q2), 共轭/1(q)
  Mux/1 -> 四元数乘法/2(Q2)
  四元数乘法/1(Q*) -> hat-s_b/1(Q1)
  共轭/1(q*) -> 四元数乘法/1(Q1)
  hat-s_b/1(Q*) -> Add/1
  太敏噪声/1(noise) -> Add/2
  Demux2/1 -> 向量模长-s_b/1(u0)
  Add/1 -> 太敏故障/1(原值)
  向量模长-s_b/1(|u|) -> Divide/2
  Demux2/2 -> 向量模长-s_b/2(u1)
  Demux2/3 -> 向量模长-s_b/3(u2)
  Divide/1 -> Dot Product/1, s_b_meas/1
  Constant/1 -> Dot Product/2
  Dot Product/1 -> Relational Operator/1
  Constant1/1 -> Relational Operator/2
  Relational Operator/1 -> valid/1
  太敏故障/1(故障值) -> Demux2/1, Divide/1

== system satellite3/姿态确定与控制系统/三轴姿态动力学子系统/姿态解算/简化互补滤波器/星敏故障/偏差故障 ==
  使能*幅度 : Gain  Gain=star_bias_on*star_bias_value
  注入时间 : Step  Time=star_bias_time  SampleTime=0
  故障值注入 : Outport
  wires:
  使能*幅度/1 -> 故障值注入/1
  注入时间/1 -> 使能*幅度/1

== system satellite3/姿态确定与控制系统/三轴姿态动力学子系统/姿态解算/简化互补滤波器/星敏故障/延迟故障 ==
  原值 : Inport
  Delay : Delay  DelayLength=star_delay_value
  Switch : Switch  Criteria=u2 > Threshold  Threshold=0.5  SaturateOnIntegerOverflow=off  InputSameDT=off
  使能 : Gain  Gain=star_delay_on
  抵消 : Sum  Inputs=|+-
  注入时间 : Step  Time=star_delay_time  SampleTime=0
  故障值注入 : Outport
  wires:
  Delay/1 -> Switch/1
  Switch/1 -> 抵消/1
  抵消/1 -> 故障值注入/1
  原值/1 -> 抵消/2, Delay/1, Switch/3
  注入时间/1 -> 使能/1
  使能/1 -> Switch/2

== system satellite3/姿态确定与控制系统/三轴姿态动力学子系统/姿态解算/简化互补滤波器/星敏故障/掉线故障 ==
  原值 : Inport
  Switch : Switch  Criteria=u2 > Threshold  Threshold=0.5  SaturateOnIntegerOverflow=off  InputSameDT=off
  Zero : Constant  Value=star_drop_value  OutDataTypeStr=Inherit: Inherit via back propagation
  使能 : Gain  Gain=star_drop_on
  抵消 : Sum  Inputs=|+-
  注入时间 : Step  Time=star_drop_time  SampleTime=0
  故障值注入 : Outport
  wires:
  使能/1 -> Switch/2
  注入时间/1 -> 使能/1
  原值/1 -> Switch/3, 抵消/2
  抵消/1 -> 故障值注入/1
  Switch/1 -> 抵消/1
  Zero/1 -> Switch/1

== system satellite3/姿态确定与控制系统/三轴姿态动力学子系统/姿态解算/简化互补滤波器/星敏故障/漂移故障 ==
  使能*幅度 : Gain  Gain=star_bias_on*star_drift_value
  注入时间 : simulink/Sources/Ramp  slope=1  start=star_drift_time  InitialOutput=0
  限幅 : Saturate  UpperLimit=star_drift_max  LowerLimit=-star_drift_max
  故障值注入 : Outport
  wires:
  限幅/1 -> 故障值注入/1
  注入时间/1 -> 使能*幅度/1
  使能*幅度/1 -> 限幅/1

== system satellite3/姿态确定与控制系统/三轴姿态动力学子系统/姿态解算/简化互补滤波器/星敏故障/锁死故障 ==
  原值 : Inport
  Switch : Switch  Criteria=u2 > Threshold  Threshold=0.5  SaturateOnIntegerOverflow=off  InputSameDT=off
  上一值 : UnitDelay  SampleTime=-1  HasFrameUpgradeWarning=on
  使能 : Gain  Gain=star_lock_on
  抵消 : Sum  Inputs=|+-
  注入时间 : Step  Time=star_lock_time  SampleTime=0
  故障值注入 : Outport
  wires:
  Switch/1 -> 抵消/1, 上一值/1
  原值/1 -> 抵消/2, Switch/3
  使能/1 -> Switch/2
  上一值/1 -> Switch/1
  抵消/1 -> 故障值注入/1
  注入时间/1 -> 使能/1

== system satellite3/姿态确定与控制系统/金字塔反作用轮组件/反作用轮组件/反作用轮1/轮力矩故障/延迟故障 ==
  原值 : Inport
  Delay : Delay  DelayLength=rw1_delay_value
  Switch : Switch  Criteria=u2 > Threshold  Threshold=0.5  SaturateOnIntegerOverflow=off  InputSameDT=off
  使能 : Gain  Gain=rw1_delay_on
  抵消 : Sum  Inputs=|+-
  注入时间 : Step  Time=rw1_delay_time  SampleTime=0
  故障值注入 : Outport
  wires:
  Delay/1 -> Switch/1
  Switch/1 -> 抵消/1
  抵消/1 -> 故障值注入/1
  原值/1 -> 抵消/2, Delay/1, Switch/3
  注入时间/1 -> 使能/1
  使能/1 -> Switch/2

== system satellite3/姿态确定与控制系统/金字塔反作用轮组件/反作用轮组件/反作用轮1/轮力矩故障/掉线故障 ==
  原值 : Inport
  Switch : Switch  Criteria=u2 > Threshold  Threshold=0.5  SaturateOnIntegerOverflow=off  InputSameDT=off
  Zero : Constant  Value=rw1_drop_value  OutDataTypeStr=Inherit: Inherit via back propagation
  使能 : Gain  Gain=rw1_drop_on
  抵消 : Sum  Inputs=|+-
  注入时间 : Step  Time=rw1_drop_time  SampleTime=0
  故障值注入 : Outport
  wires:
  使能/1 -> Switch/2
  注入时间/1 -> 使能/1
  原值/1 -> Switch/3, 抵消/2
  抵消/1 -> 故障值注入/1
  Switch/1 -> 抵消/1
  Zero/1 -> Switch/1

== system satellite3/姿态确定与控制系统/金字塔反作用轮组件/反作用轮组件/反作用轮1/轮力矩故障/迟缓故障 ==
  原值 : Inport
  Switch : Switch  Criteria=u2 > Threshold  Threshold=0.5  SaturateOnIntegerOverflow=off  InputSameDT=off
  使能 : Gain  Gain=rw1_slow_on
  幅度 : RateLimiter  RisingSlewLimit=rw1_slow_value  FallingSlewLimit=-rw1_slow_value  SampleTimeMode=inherited
  抵消 : Sum  Inputs=|+-
  注入时间 : Step  Time=rw1_slow_time  SampleTime=0
  故障值注入 : Outport
  wires:
  幅度/1 -> Switch/1
  Switch/1 -> 抵消/1
  抵消/1 -> 故障值注入/1
  原值/1 -> 抵消/2, 幅度/1, Switch/3
  注入时间/1 -> 使能/1
  使能/1 -> Switch/2

== system satellite3/姿态确定与控制系统/金字塔反作用轮组件/反作用轮组件/反作用轮1/轮力矩故障/退化故障 ==
  原值 : Inport
  Switch : Switch  Criteria=u2 > Threshold  Threshold=0.5  SaturateOnIntegerOverflow=off  InputSameDT=off
  使能 : Gain  Gain=rw1_deg_on
  幅度 : Gain  Gain=rw1_deg_value
  抵消 : Sum  Inputs=|+-
  注入时间 : Step  Time=rw1_deg_time  SampleTime=0
  故障值注入 : Outport
  wires:
  Switch/1 -> 抵消/1
  原值/1 -> 抵消/2, 幅度/1, Switch/3
  使能/1 -> Switch/2
  抵消/1 -> 故障值注入/1
  注入时间/1 -> 使能/1
  幅度/1 -> Switch/1

== system satellite3/姿态确定与控制系统/金字塔反作用轮组件/反作用轮组件/反作用轮1/轮力矩故障/锁死故障 ==
  原值 : Inport
  Switch : Switch  Criteria=u2 > Threshold  Threshold=0.5  SaturateOnIntegerOverflow=off  InputSameDT=off
  上一值 : UnitDelay  SampleTime=-1  HasFrameUpgradeWarning=on
  使能 : Gain  Gain=rw1_lock_on
  抵消 : Sum  Inputs=|+-
  注入时间 : Step  Time=rw1_lock_time  SampleTime=0
  故障值注入 : Outport
  wires:
  Switch/1 -> 抵消/1, 上一值/1
  原值/1 -> 抵消/2, Switch/3
  使能/1 -> Switch/2
  上一值/1 -> Switch/1
  抵消/1 -> 故障值注入/1
  注入时间/1 -> 使能/1

== system satellite3/姿态确定与控制系统/金字塔反作用轮组件/反作用轮组件/反作用轮1/轮力矩故障/饱和故障 ==
  原值 : Inport
  Saturation : Saturate  UpperLimit=rw1_sat_value*T_max  LowerLimit=-rw1_sat_value*T_max
  Switch : Switch  Criteria=u2 > Threshold  Threshold=0.5  SaturateOnIntegerOverflow=off  InputSameDT=off
  使能 : Gain  Gain=rw1_sat_on
  抵消 : Sum  Inputs=|+-
  注入时间 : Step  Time=rw1_sat_time  SampleTime=0
  故障值注入 : Outport
  wires:
  使能/1 -> Switch/2
  注入时间/1 -> 使能/1
  原值/1 -> 抵消/2, Saturation/1, Switch/3
  抵消/1 -> 故障值注入/1
  Switch/1 -> 抵消/1
  Saturation/1 -> Switch/1

== system satellite3/姿态确定与控制系统/金字塔反作用轮组件/反作用轮组件/反作用轮1/轮摩擦故障/乘性故障 ==
  原值 : Inport
  Switch : Switch  Criteria=u2 > Threshold  Threshold=0.5  SaturateOnIntegerOverflow=off  InputSameDT=off
  使能 : Gain  Gain=rw1_fric_on
  幅度 : Gain  Gain=rw1_fric_value
  抵消 : Sum  Inputs=|+-
  注入时间 : Step  Time=rw1_fric_time  SampleTime=0
  故障值注入 : Outport
  wires:
  Switch/1 -> 抵消/1
  原值/1 -> 抵消/2, 幅度/1, Switch/3
  使能/1 -> Switch/2
  抵消/1 -> 故障值注入/1
  注入时间/1 -> 使能/1
  幅度/1 -> Switch/1

== system satellite3/姿态确定与控制系统/金字塔反作用轮组件/反作用轮组件/反作用轮1/轮摩擦故障/偏差故障 ==
  使能*幅度 : Gain  Gain=rw1_bias_on*rw1_bias_value
  注入时间 : Step  Time=rw1_bias_time  SampleTime=0
  故障值注入 : Outport
  wires:
  使能*幅度/1 -> 故障值注入/1
  注入时间/1 -> 使能*幅度/1

== system satellite3/姿态确定与控制系统/金字塔反作用轮组件/反作用轮组件/反作用轮2/轮力矩故障/延迟故障 ==
  原值 : Inport
  Delay : Delay  DelayLength=rw2_delay_value
  Switch : Switch  Criteria=u2 > Threshold  Threshold=0.5  SaturateOnIntegerOverflow=off  InputSameDT=off
  使能 : Gain  Gain=rw2_delay_on
  抵消 : Sum  Inputs=|+-
  注入时间 : Step  Time=rw2_delay_time  SampleTime=0
  故障值注入 : Outport
  wires:
  使能/1 -> Switch/2
  注入时间/1 -> 使能/1
  原值/1 -> Switch/3, Delay/1, 抵消/2
  抵消/1 -> 故障值注入/1
  Switch/1 -> 抵消/1
  Delay/1 -> Switch/1

== system satellite3/姿态确定与控制系统/金字塔反作用轮组件/反作用轮组件/反作用轮2/轮力矩故障/掉线故障 ==
  原值 : Inport
  Switch : Switch  Criteria=u2 > Threshold  Threshold=0.5  SaturateOnIntegerOverflow=off  InputSameDT=off
  Zero : Constant  Value=rw2_drop_value  OutDataTypeStr=Inherit: Inherit via back propagation
  使能 : Gain  Gain=rw2_drop_on
  抵消 : Sum  Inputs=|+-
  注入时间 : Step  Time=rw2_drop_time  SampleTime=0
  故障值注入 : Outport
  wires:
  Zero/1 -> Switch/1
  Switch/1 -> 抵消/1
  抵消/1 -> 故障值注入/1
  原值/1 -> 抵消/2, Switch/3
  注入时间/1 -> 使能/1
  使能/1 -> Switch/2

== system satellite3/姿态确定与控制系统/金字塔反作用轮组件/反作用轮组件/反作用轮2/轮力矩故障/迟缓故障 ==
  原值 : Inport
  Switch : Switch  Criteria=u2 > Threshold  Threshold=0.5  SaturateOnIntegerOverflow=off  InputSameDT=off
  使能 : Gain  Gain=rw2_slow_on
  幅度 : RateLimiter  RisingSlewLimit=rw2_slow_value  FallingSlewLimit=-rw2_slow_value  SampleTimeMode=inherited
  抵消 : Sum  Inputs=|+-
  注入时间 : Step  Time=rw2_slow_time  SampleTime=0
  故障值注入 : Outport
  wires:
  使能/1 -> Switch/2
  注入时间/1 -> 使能/1
  原值/1 -> Switch/3, 幅度/1, 抵消/2
  抵消/1 -> 故障值注入/1
  Switch/1 -> 抵消/1
  幅度/1 -> Switch/1

== system satellite3/姿态确定与控制系统/金字塔反作用轮组件/反作用轮组件/反作用轮2/轮力矩故障/退化故障 ==
  原值 : Inport
  Switch : Switch  Criteria=u2 > Threshold  Threshold=0.5  SaturateOnIntegerOverflow=off  InputSameDT=off
  使能 : Gain  Gain=rw2_deg_on
  幅度 : Gain  Gain=rw2_deg_value
  抵消 : Sum  Inputs=|+-
  注入时间 : Step  Time=rw2_deg_time  SampleTime=0
  故障值注入 : Outport
  wires:
  幅度/1 -> Switch/1
  注入时间/1 -> 使能/1
  抵消/1 -> 故障值注入/1
  使能/1 -> Switch/2
  原值/1 -> Switch/3, 幅度/1, 抵消/2
  Switch/1 -> 抵消/1

== system satellite3/姿态确定与控制系统/金字塔反作用轮组件/反作用轮组件/反作用轮2/轮力矩故障/锁死故障 ==
  原值 : Inport
  Switch : Switch  Criteria=u2 > Threshold  Threshold=0.5  SaturateOnIntegerOverflow=off  InputSameDT=off
  上一值 : UnitDelay  SampleTime=-1  HasFrameUpgradeWarning=on
  使能 : Gain  Gain=rw2_lock_on
  抵消 : Sum  Inputs=|+-
  注入时间 : Step  Time=rw2_lock_time  SampleTime=0
  故障值注入 : Outport
  wires:
  注入时间/1 -> 使能/1
  抵消/1 -> 故障值注入/1
  上一值/1 -> Switch/1
  使能/1 -> Switch/2
  原值/1 -> Switch/3, 抵消/2
  Switch/1 -> 上一值/1, 抵消/1

== system satellite3/姿态确定与控制系统/金字塔反作用轮组件/反作用轮组件/反作用轮2/轮力矩故障/饱和故障 ==
  原值 : Inport
  Saturation : Saturate  UpperLimit=rw2_sat_value*T_max  LowerLimit=-rw2_sat_value*T_max
  Switch : Switch  Criteria=u2 > Threshold  Threshold=0.5  SaturateOnIntegerOverflow=off  InputSameDT=off
  使能 : Gain  Gain=rw2_sat_on
  抵消 : Sum  Inputs=|+-
  注入时间 : Step  Time=rw2_sat_time  SampleTime=0
  故障值注入 : Outport
  wires:
  Saturation/1 -> Switch/1
  Switch/1 -> 抵消/1
  抵消/1 -> 故障值注入/1
  原值/1 -> Switch/3, Saturation/1, 抵消/2
  注入时间/1 -> 使能/1
  使能/1 -> Switch/2

== system satellite3/姿态确定与控制系统/金字塔反作用轮组件/反作用轮组件/反作用轮2/轮摩擦故障/乘性故障 ==
  原值 : Inport
  Switch : Switch  Criteria=u2 > Threshold  Threshold=0.5  SaturateOnIntegerOverflow=off  InputSameDT=off
  使能 : Gain  Gain=rw2_fric_on
  幅度 : Gain  Gain=rw2_fric_value
  抵消 : Sum  Inputs=|+-
  注入时间 : Step  Time=rw2_fric_time  SampleTime=0
  故障值注入 : Outport
  wires:
  Switch/1 -> 抵消/1
  原值/1 -> 抵消/2, 幅度/1, Switch/3
  使能/1 -> Switch/2
  抵消/1 -> 故障值注入/1
  注入时间/1 -> 使能/1
  幅度/1 -> Switch/1

== system satellite3/姿态确定与控制系统/金字塔反作用轮组件/反作用轮组件/反作用轮2/轮摩擦故障/偏差故障 ==
  使能*幅度 : Gain  Gain=rw2_bias_on*rw2_bias_value
  注入时间 : Step  Time=rw2_bias_time  SampleTime=0
  故障值注入 : Outport
  wires:
  使能*幅度/1 -> 故障值注入/1
  注入时间/1 -> 使能*幅度/1

== system satellite3/姿态确定与控制系统/金字塔反作用轮组件/反作用轮组件/反作用轮3/轮力矩故障/延迟故障 ==
  原值 : Inport
  Delay : Delay  DelayLength=rw3_delay_value
  Switch : Switch  Criteria=u2 > Threshold  Threshold=0.5  SaturateOnIntegerOverflow=off  InputSameDT=off
  使能 : Gain  Gain=rw3_delay_on
  抵消 : Sum  Inputs=|+-
  注入时间 : Step  Time=rw3_delay_time  SampleTime=0
  故障值注入 : Outport
  wires:
  Delay/1 -> Switch/1
  Switch/1 -> 抵消/1
  抵消/1 -> 故障值注入/1
  原值/1 -> 抵消/2, Delay/1, Switch/3
  注入时间/1 -> 使能/1
  使能/1 -> Switch/2

== system satellite3/姿态确定与控制系统/金字塔反作用轮组件/反作用轮组件/反作用轮3/轮力矩故障/掉线故障 ==
  原值 : Inport
  Switch : Switch  Criteria=u2 > Threshold  Threshold=0.5  SaturateOnIntegerOverflow=off  InputSameDT=off
  Zero : Constant  Value=rw3_drop_value  OutDataTypeStr=Inherit: Inherit via back propagation
  使能 : Gain  Gain=rw3_drop_on
  抵消 : Sum  Inputs=|+-
  注入时间 : Step  Time=rw3_drop_time  SampleTime=0
  故障值注入 : Outport
  wires:
  使能/1 -> Switch/2
  注入时间/1 -> 使能/1
  原值/1 -> Switch/3, 抵消/2
  抵消/1 -> 故障值注入/1
  Switch/1 -> 抵消/1
  Zero/1 -> Switch/1

== system satellite3/姿态确定与控制系统/金字塔反作用轮组件/反作用轮组件/反作用轮3/轮力矩故障/迟缓故障 ==
  原值 : Inport
  Switch : Switch  Criteria=u2 > Threshold  Threshold=0.5  SaturateOnIntegerOverflow=off  InputSameDT=off
  使能 : Gain  Gain=rw3_slow_on
  幅度 : RateLimiter  RisingSlewLimit=rw3_slow_value  FallingSlewLimit=-rw3_slow_value  SampleTimeMode=inherited
  抵消 : Sum  Inputs=|+-
  注入时间 : Step  Time=rw3_slow_time  SampleTime=0
  故障值注入 : Outport
  wires:
  幅度/1 -> Switch/1
  Switch/1 -> 抵消/1
  抵消/1 -> 故障值注入/1
  原值/1 -> 抵消/2, 幅度/1, Switch/3
  注入时间/1 -> 使能/1
  使能/1 -> Switch/2

== system satellite3/姿态确定与控制系统/金字塔反作用轮组件/反作用轮组件/反作用轮3/轮力矩故障/退化故障 ==
  原值 : Inport
  Switch : Switch  Criteria=u2 > Threshold  Threshold=0.5  SaturateOnIntegerOverflow=off  InputSameDT=off
  使能 : Gain  Gain=rw3_deg_on
  幅度 : Gain  Gain=rw3_deg_value
  抵消 : Sum  Inputs=|+-
  注入时间 : Step  Time=rw3_deg_time  SampleTime=0
  故障值注入 : Outport
  wires:
  Switch/1 -> 抵消/1
  原值/1 -> 抵消/2, 幅度/1, Switch/3
  使能/1 -> Switch/2
  抵消/1 -> 故障值注入/1
  注入时间/1 -> 使能/1
  幅度/1 -> Switch/1

== system satellite3/姿态确定与控制系统/金字塔反作用轮组件/反作用轮组件/反作用轮3/轮力矩故障/锁死故障 ==
  原值 : Inport
  Switch : Switch  Criteria=u2 > Threshold  Threshold=0.5  SaturateOnIntegerOverflow=off  InputSameDT=off
  上一值 : UnitDelay  SampleTime=-1  HasFrameUpgradeWarning=on
  使能 : Gain  Gain=rw3_lock_on
  抵消 : Sum  Inputs=|+-
  注入时间 : Step  Time=rw3_lock_time  SampleTime=0
  故障值注入 : Outport
  wires:
  Switch/1 -> 抵消/1, 上一值/1
  原值/1 -> 抵消/2, Switch/3
  使能/1 -> Switch/2
  上一值/1 -> Switch/1
  抵消/1 -> 故障值注入/1
  注入时间/1 -> 使能/1

== system satellite3/姿态确定与控制系统/金字塔反作用轮组件/反作用轮组件/反作用轮3/轮力矩故障/饱和故障 ==
  原值 : Inport
  Saturation : Saturate  UpperLimit=rw3_sat_value*T_max  LowerLimit=-rw3_sat_value*T_max
  Switch : Switch  Criteria=u2 > Threshold  Threshold=0.5  SaturateOnIntegerOverflow=off  InputSameDT=off
  使能 : Gain  Gain=rw3_sat_on
  抵消 : Sum  Inputs=|+-
  注入时间 : Step  Time=rw3_sat_time  SampleTime=0
  故障值注入 : Outport
  wires:
  使能/1 -> Switch/2
  注入时间/1 -> 使能/1
  原值/1 -> 抵消/2, Saturation/1, Switch/3
  抵消/1 -> 故障值注入/1
  Switch/1 -> 抵消/1
  Saturation/1 -> Switch/1

== system satellite3/姿态确定与控制系统/金字塔反作用轮组件/反作用轮组件/反作用轮3/轮摩擦故障/乘性故障 ==
  原值 : Inport
  Switch : Switch  Criteria=u2 > Threshold  Threshold=0.5  SaturateOnIntegerOverflow=off  InputSameDT=off
  使能 : Gain  Gain=rw3_fric_on
  幅度 : Gain  Gain=rw3_fric_value
  抵消 : Sum  Inputs=|+-
  注入时间 : Step  Time=rw3_fric_time  SampleTime=0
  故障值注入 : Outport
  wires:
  Switch/1 -> 抵消/1
  原值/1 -> 抵消/2, 幅度/1, Switch/3
  使能/1 -> Switch/2
  抵消/1 -> 故障值注入/1
  注入时间/1 -> 使能/1
  幅度/1 -> Switch/1

== system satellite3/姿态确定与控制系统/金字塔反作用轮组件/反作用轮组件/反作用轮3/轮摩擦故障/偏差故障 ==
  使能*幅度 : Gain  Gain=rw3_bias_on*rw3_bias_value
  注入时间 : Step  Time=rw3_bias_time  SampleTime=0
  故障值注入 : Outport
  wires:
  使能*幅度/1 -> 故障值注入/1
  注入时间/1 -> 使能*幅度/1

== system satellite3/姿态确定与控制系统/金字塔反作用轮组件/反作用轮组件/反作用轮4/轮力矩故障/延迟故障 ==
  原值 : Inport
  Delay : Delay  DelayLength=rw4_delay_value
  Switch : Switch  Criteria=u2 > Threshold  Threshold=0.5  SaturateOnIntegerOverflow=off  InputSameDT=off
  使能 : Gain  Gain=rw4_delay_on
  抵消 : Sum  Inputs=|+-
  注入时间 : Step  Time=rw4_delay_time  SampleTime=0
  故障值注入 : Outport
  wires:
  使能/1 -> Switch/2
  注入时间/1 -> 使能/1
  原值/1 -> Switch/3, Delay/1, 抵消/2
  抵消/1 -> 故障值注入/1
  Switch/1 -> 抵消/1
  Delay/1 -> Switch/1

== system satellite3/姿态确定与控制系统/金字塔反作用轮组件/反作用轮组件/反作用轮4/轮力矩故障/掉线故障 ==
  原值 : Inport
  Switch : Switch  Criteria=u2 > Threshold  Threshold=0.5  SaturateOnIntegerOverflow=off  InputSameDT=off
  Zero : Constant  Value=rw4_drop_value  OutDataTypeStr=Inherit: Inherit via back propagation
  使能 : Gain  Gain=rw4_drop_on
  抵消 : Sum  Inputs=|+-
  注入时间 : Step  Time=rw4_drop_time  SampleTime=0
  故障值注入 : Outport
  wires:
  Zero/1 -> Switch/1
  Switch/1 -> 抵消/1
  抵消/1 -> 故障值注入/1
  原值/1 -> 抵消/2, Switch/3
  注入时间/1 -> 使能/1
  使能/1 -> Switch/2

== system satellite3/姿态确定与控制系统/金字塔反作用轮组件/反作用轮组件/反作用轮4/轮力矩故障/迟缓故障 ==
  原值 : Inport
  Switch : Switch  Criteria=u2 > Threshold  Threshold=0.5  SaturateOnIntegerOverflow=off  InputSameDT=off
  使能 : Gain  Gain=rw4_slow_on
  幅度 : RateLimiter  RisingSlewLimit=rw4_slow_value  FallingSlewLimit=-rw4_slow_value  SampleTimeMode=inherited
  抵消 : Sum  Inputs=|+-
  注入时间 : Step  Time=rw4_slow_time  SampleTime=0
  故障值注入 : Outport
  wires:
  使能/1 -> Switch/2
  注入时间/1 -> 使能/1
  原值/1 -> Switch/3, 幅度/1, 抵消/2
  抵消/1 -> 故障值注入/1
  Switch/1 -> 抵消/1
  幅度/1 -> Switch/1

== system satellite3/姿态确定与控制系统/金字塔反作用轮组件/反作用轮组件/反作用轮4/轮力矩故障/退化故障 ==
  原值 : Inport
  Switch : Switch  Criteria=u2 > Threshold  Threshold=0.5  SaturateOnIntegerOverflow=off  InputSameDT=off
  使能 : Gain  Gain=rw4_deg_on
  幅度 : Gain  Gain=rw4_deg_value
  抵消 : Sum  Inputs=|+-
  注入时间 : Step  Time=rw4_deg_time  SampleTime=0
  故障值注入 : Outport
  wires:
  幅度/1 -> Switch/1
  注入时间/1 -> 使能/1
  抵消/1 -> 故障值注入/1
  使能/1 -> Switch/2
  原值/1 -> Switch/3, 幅度/1, 抵消/2
  Switch/1 -> 抵消/1

== system satellite3/姿态确定与控制系统/金字塔反作用轮组件/反作用轮组件/反作用轮4/轮力矩故障/锁死故障 ==
  原值 : Inport
  Switch : Switch  Criteria=u2 > Threshold  Threshold=0.5  SaturateOnIntegerOverflow=off  InputSameDT=off
  上一值 : UnitDelay  SampleTime=-1  HasFrameUpgradeWarning=on
  使能 : Gain  Gain=rw4_lock_on
  抵消 : Sum  Inputs=|+-
  注入时间 : Step  Time=rw4_lock_time  SampleTime=0
  故障值注入 : Outport
  wires:
  注入时间/1 -> 使能/1
  抵消/1 -> 故障值注入/1
  上一值/1 -> Switch/1
  使能/1 -> Switch/2
  原值/1 -> Switch/3, 抵消/2
  Switch/1 -> 上一值/1, 抵消/1

== system satellite3/姿态确定与控制系统/金字塔反作用轮组件/反作用轮组件/反作用轮4/轮力矩故障/饱和故障 ==
  原值 : Inport
  Saturation : Saturate  UpperLimit=rw4_sat_value*T_max  LowerLimit=-rw4_sat_value*T_max
  Switch : Switch  Criteria=u2 > Threshold  Threshold=0.5  SaturateOnIntegerOverflow=off  InputSameDT=off
  使能 : Gain  Gain=rw4_sat_on
  抵消 : Sum  Inputs=|+-
  注入时间 : Step  Time=rw4_sat_time  SampleTime=0
  故障值注入 : Outport
  wires:
  Saturation/1 -> Switch/1
  Switch/1 -> 抵消/1
  抵消/1 -> 故障值注入/1
  原值/1 -> Switch/3, Saturation/1, 抵消/2
  注入时间/1 -> 使能/1
  使能/1 -> Switch/2

== system satellite3/姿态确定与控制系统/金字塔反作用轮组件/反作用轮组件/反作用轮4/轮摩擦故障/乘性故障 ==
  原值 : Inport
  Switch : Switch  Criteria=u2 > Threshold  Threshold=0.5  SaturateOnIntegerOverflow=off  InputSameDT=off
  使能 : Gain  Gain=rw4_fric_on
  幅度 : Gain  Gain=rw4_fric_value
  抵消 : Sum  Inputs=|+-
  注入时间 : Step  Time=rw4_fric_time  SampleTime=0
  故障值注入 : Outport
  wires:
  Switch/1 -> 抵消/1
  原值/1 -> 抵消/2, 幅度/1, Switch/3
  使能/1 -> Switch/2
  抵消/1 -> 故障值注入/1
  注入时间/1 -> 使能/1
  幅度/1 -> Switch/1

== system satellite3/姿态确定与控制系统/金字塔反作用轮组件/反作用轮组件/反作用轮4/轮摩擦故障/偏差故障 ==
  使能*幅度 : Gain  Gain=rw4_bias_on*rw4_bias_value
  注入时间 : Step  Time=rw4_bias_time  SampleTime=0
  故障值注入 : Outport
  wires:
  使能*幅度/1 -> 故障值注入/1
  注入时间/1 -> 使能*幅度/1

== system satellite3/电源子系统/太阳能板/太阳板/入射角余弦/余弦夹角/向量模长-r1 ==
  u1 : Inport
  u2 : Inport  Port=2
  u3 : Inport  Port=3
  Add : Sum  Inputs=+++
  Sqrt : Sqrt
  Square : Math  Operator=square
  Square1 : Math  Operator=square
  Square2 : Math  Operator=square
  |u| : Outport
  wires:
  Sqrt/1 -> |u|/1
  Add/1 -> Sqrt/1
  Square2/1 -> Add/3
  Square1/1 -> Add/2
  Square/1 -> Add/1
  u3/1 -> Square2/1
  u2/1 -> Square1/1
  u1/1 -> Square/1

== system satellite3/电源子系统/太阳能板/太阳板/入射角余弦/余弦夹角/向量模长-r2 ==
  u1 : Inport
  u2 : Inport  Port=2
  u3 : Inport  Port=3
  Add : Sum  Inputs=+++
  Sqrt : Sqrt
  Square : Math  Operator=square
  Square1 : Math  Operator=square
  Square2 : Math  Operator=square
  |u| : Outport
  wires:
  u1/1 -> Square/1
  u2/1 -> Square1/1
  u3/1 -> Square2/1
  Square/1 -> Add/1
  Square1/1 -> Add/2
  Square2/1 -> Add/3
  Add/1 -> Sqrt/1
  Sqrt/1 -> |u|/1

== system satellite3/姿态确定与控制系统/三轴姿态动力学子系统/姿态解算/简化互补滤波器/太敏&地敏/地敏测量/hat-s_b ==
  Q1 : Inport
  Q2 : Inport  Port=2
  Add : Sum  Inputs=3
  Cross Product : matrix_library/Cross Product
  Demux : Demux
  Demux1 : Demux
  Mux1 : Mux  Inputs=3
  Mux2 : Mux  Inputs=3
  Product : Product  Inputs=*/
  Product1 : Product
  Product2 : Product
  向量模长-T : Subsystem
  hat_r_b : Outport
  wires:
  Demux1/4 -> Mux2/3
  Demux1/3 -> Mux2/2
  Demux1/2 -> Mux2/1
  Demux/4 -> Mux1/3
  Demux/3 -> Mux1/2
  Demux/2 -> Mux1/1
  Cross Product/1 -> Add/3
  Product1/1 -> Add/1
  Product2/1 -> Add/2
  Mux2/1 -> Product1/2, Cross Product/2
  Demux1/1 -> Product2/1
  Mux1/1 -> Product2/2, Cross Product/1
  Demux/1 -> Product1/1
  Q2/1 -> Demux1/1
  Q1/1 -> Demux/1
  Add/1 -> Product/1, 向量模长-T/1(u)
  Product/1 -> hat_r_b/1
  向量模长-T/1(|u|) -> Product/2

== system satellite3/姿态确定与控制系统/三轴姿态动力学子系统/姿态解算/简化互补滤波器/太敏&地敏/地敏测量/共轭 ==
  q : Inport
  -qd1 : Gain  Gain=-1
  -qd2 : Gain  Gain=-1
  -qd3 : Gain  Gain=-1
  Demux : Demux
  Mux : Mux
  q* : Outport
  wires:
  q/1 -> Demux/1
  Mux/1 -> q*/1
  Demux/1 -> Mux/1
  Demux/2 -> -qd1/1
  -qd1/1 -> Mux/2
  Demux/3 -> -qd2/1
  -qd2/1 -> Mux/3
  Demux/4 -> -qd3/1
  -qd3/1 -> Mux/4

== system satellite3/姿态确定与控制系统/三轴姿态动力学子系统/姿态解算/简化互补滤波器/太敏&地敏/地敏测量/向量模长-s_b ==
  u0 : Inport
  u1 : Inport  Port=2
  u2 : Inport  Port=3
  Add : Sum  Inputs=3
  Sqrt : Sqrt
  Square : Math  Operator=square
  Square1 : Math  Operator=square
  Square2 : Math  Operator=square
  |u| : Outport
  wires:
  u0/1 -> Square/1
  u1/1 -> Square1/1
  u2/1 -> Square2/1
  Square/1 -> Add/1
  Square1/1 -> Add/2
  Square2/1 -> Add/3
  Add/1 -> Sqrt/1
  Sqrt/1 -> |u|/1

== system satellite3/姿态确定与控制系统/三轴姿态动力学子系统/姿态解算/简化互补滤波器/太敏&地敏/地敏测量/四元数乘法 ==
  Q1 : Inport
  Q2 : Inport  Port=2
  Add : Sum  Inputs=3
  Cross Product : matrix_library/Cross Product
  Demux : Demux
  Demux1 : Demux
  Dot Product : DotProduct  OutDataTypeStr=Inherit: Inherit via internal rule
  Mux : Mux  Inputs=2
  Mux1 : Mux  Inputs=3
  Mux2 : Mux  Inputs=3
  Product : Product
  Product1 : Product
  Product2 : Product
  Sum : Sum  Inputs=|+-
  Q* : Outport
  wires:
  Q1/1 -> Demux/1
  Q2/1 -> Demux1/1
  Mux/1 -> Q*/1
  Product/1 -> Sum/1
  Demux/1 -> Product1/1, Product/1
  Mux1/1 -> Dot Product/1, Cross Product/1, Product2/2
  Demux1/1 -> Product2/1, Product/2
  Mux2/1 -> Cross Product/2, Dot Product/2, Product1/2
  Sum/1 -> Mux/1
  Dot Product/1 -> Sum/2
  Product2/1 -> Add/2
  Product1/1 -> Add/1
  Cross Product/1 -> Add/3
  Add/1 -> Mux/2
  Demux/2 -> Mux1/1
  Demux/3 -> Mux1/2
  Demux/4 -> Mux1/3
  Demux1/2 -> Mux2/1
  Demux1/3 -> Mux2/2
  Demux1/4 -> Mux2/3

== system satellite3/姿态确定与控制系统/三轴姿态动力学子系统/姿态解算/简化互补滤波器/太敏&地敏/地敏预测/hat-s_b ==
  Q1 : Inport
  Q2 : Inport  Port=2
  Add : Sum  Inputs=3
  Cross Product : matrix_library/Cross Product
  Demux : Demux
  Demux1 : Demux
  Mux1 : Mux  Inputs=3
  Mux2 : Mux  Inputs=3
  Product : Product  Inputs=*/
  Product1 : Product
  Product2 : Product
  向量模长-T : Subsystem
  hat_r_b : Outport
  wires:
  Demux1/4 -> Mux2/3
  Demux1/3 -> Mux2/2
  Demux1/2 -> Mux2/1
  Demux/4 -> Mux1/3
  Demux/3 -> Mux1/2
  Demux/2 -> Mux1/1
  Cross Product/1 -> Add/3
  Product1/1 -> Add/1
  Product2/1 -> Add/2
  Mux2/1 -> Product1/2, Cross Product/2
  Demux1/1 -> Product2/1
  Mux1/1 -> Product2/2, Cross Product/1
  Demux/1 -> Product1/1
  Q2/1 -> Demux1/1
  Q1/1 -> Demux/1
  Add/1 -> Product/1, 向量模长-T/1(u)
  Product/1 -> hat_r_b/1
  向量模长-T/1(|u|) -> Product/2

== system satellite3/姿态确定与控制系统/三轴姿态动力学子系统/姿态解算/简化互补滤波器/太敏&地敏/地敏预测/共轭 ==
  q : Inport
  -qd1 : Gain  Gain=-1
  -qd2 : Gain  Gain=-1
  -qd3 : Gain  Gain=-1
  Demux : Demux
  Mux : Mux
  q* : Outport
  wires:
  q/1 -> Demux/1
  Mux/1 -> q*/1
  Demux/1 -> Mux/1
  Demux/2 -> -qd1/1
  -qd1/1 -> Mux/2
  Demux/3 -> -qd2/1
  -qd2/1 -> Mux/3
  Demux/4 -> -qd3/1
  -qd3/1 -> Mux/4

== system satellite3/姿态确定与控制系统/三轴姿态动力学子系统/姿态解算/简化互补滤波器/太敏&地敏/地敏预测/向量模长-s_b ==
  u0 : Inport
  u1 : Inport  Port=2
  u2 : Inport  Port=3
  Add : Sum  Inputs=3
  Sqrt : Sqrt
  Square : Math  Operator=square
  Square1 : Math  Operator=square
  Square2 : Math  Operator=square
  |u| : Outport
  wires:
  u0/1 -> Square/1
  u1/1 -> Square1/1
  u2/1 -> Square2/1
  Square/1 -> Add/1
  Square1/1 -> Add/2
  Square2/1 -> Add/3
  Add/1 -> Sqrt/1
  Sqrt/1 -> |u|/1

== system satellite3/姿态确定与控制系统/三轴姿态动力学子系统/姿态解算/简化互补滤波器/太敏&地敏/地敏预测/四元数乘法 ==
  Q1 : Inport
  Q2 : Inport  Port=2
  Add : Sum  Inputs=3
  Cross Product : matrix_library/Cross Product
  Demux : Demux
  Demux1 : Demux
  Dot Product : DotProduct  OutDataTypeStr=Inherit: Inherit via internal rule
  Mux : Mux  Inputs=2
  Mux1 : Mux  Inputs=3
  Mux2 : Mux  Inputs=3
  Product : Product
  Product1 : Product
  Product2 : Product
  Sum : Sum  Inputs=|+-
  Q* : Outport
  wires:
  Q1/1 -> Demux/1
  Q2/1 -> Demux1/1
  Mux/1 -> Q*/1
  Product/1 -> Sum/1
  Demux/1 -> Product1/1, Product/1
  Mux1/1 -> Dot Product/1, Cross Product/1, Product2/2
  Demux1/1 -> Product2/1, Product/2
  Mux2/1 -> Cross Product/2, Dot Product/2, Product1/2
  Sum/1 -> Mux/1
  Dot Product/1 -> Sum/2
  Product2/1 -> Add/2
  Product1/1 -> Add/1
  Cross Product/1 -> Add/3
  Add/1 -> Mux/2
  Demux/2 -> Mux1/1
  Demux/3 -> Mux1/2
  Demux/4 -> Mux1/3
  Demux1/2 -> Mux2/1
  Demux1/3 -> Mux2/2
  Demux1/4 -> Mux2/3

== system satellite3/姿态确定与控制系统/三轴姿态动力学子系统/姿态解算/简化互补滤波器/太敏&地敏/地敏预测/地敏噪声 ==
  note: 先用正弦伪噪声，再考虑换成随机噪声
  1 : simulink/Sources/Band-Limited White Noise  Cov=[0.1]  Ts=0.1  seed=[23341]
  Mux : Mux  Inputs=3
  Sine Wave : Sin  Amplitude=sigma_sun  Frequency=2*pi*1  SampleTime=0
  Sine Wave1 : Sin  Amplitude=sigma_sun  Frequency=2*pi*1  SampleTime=0
  Sine Wave2 : Sin  Amplitude=sigma_sun  Frequency=2*pi*1  SampleTime=0
  noise : Outport
  wires:
  Sine Wave/1 -> Mux/1
  Mux/1 -> noise/1
  Sine Wave1/1 -> Mux/2
  Sine Wave2/1 -> Mux/3

== system satellite3/姿态确定与控制系统/三轴姿态动力学子系统/姿态解算/简化互补滤波器/太敏&地敏/太敏测量/hat-s_b ==
  Q1 : Inport
  Q2 : Inport  Port=2
  Add : Sum  Inputs=3
  Cross Product : matrix_library/Cross Product
  Demux : Demux
  Demux1 : Demux
  Mux1 : Mux  Inputs=3
  Mux2 : Mux  Inputs=3
  Product1 : Product
  Product2 : Product
  Q* : Outport
  wires:
  Add/1 -> Q*/1
  Q1/1 -> Demux/1
  Q2/1 -> Demux1/1
  Demux/1 -> Product1/1
  Mux1/1 -> Cross Product/1, Product2/2
  Demux1/1 -> Product2/1
  Mux2/1 -> Cross Product/2, Product1/2
  Product2/1 -> Add/2
  Product1/1 -> Add/1
  Cross Product/1 -> Add/3
  Demux/2 -> Mux1/1
  Demux/3 -> Mux1/2
  Demux/4 -> Mux1/3
  Demux1/2 -> Mux2/1
  Demux1/3 -> Mux2/2
  Demux1/4 -> Mux2/3

== system satellite3/姿态确定与控制系统/三轴姿态动力学子系统/姿态解算/简化互补滤波器/太敏&地敏/太敏测量/共轭 ==
  q : Inport
  -qd1 : Gain  Gain=-1
  -qd2 : Gain  Gain=-1
  -qd3 : Gain  Gain=-1
  Demux : Demux
  Mux : Mux
  q* : Outport
  wires:
  -qd3/1 -> Mux/4
  Demux/4 -> -qd3/1
  -qd2/1 -> Mux/3
  Demux/3 -> -qd2/1
  -qd1/1 -> Mux/2
  Demux/2 -> -qd1/1
  Demux/1 -> Mux/1
  Mux/1 -> q*/1
  q/1 -> Demux/1

== system satellite3/姿态确定与控制系统/三轴姿态动力学子系统/姿态解算/简化互补滤波器/太敏&地敏/太敏测量/向量模长-s_b ==
  u0 : Inport
  u1 : Inport  Port=2
  u2 : Inport  Port=3
  Add : Sum  Inputs=3
  Sqrt : Sqrt
  Square : Math  Operator=square
  Square1 : Math  Operator=square
  Square2 : Math  Operator=square
  |u| : Outport
  wires:
  Sqrt/1 -> |u|/1
  Add/1 -> Sqrt/1
  Square2/1 -> Add/3
  Square1/1 -> Add/2
  Square/1 -> Add/1
  u2/1 -> Square2/1
  u1/1 -> Square1/1
  u0/1 -> Square/1
